simulink model "untitled"  (R2025a)
settings: Solver=VariableStepAuto  StartTime=0.0  StopTime=10.0  RelTol=1e-3
libraries: slpidlib x1
settings Model: Creator=MTMTAD006  LastModifiedBy=MTMTAD006

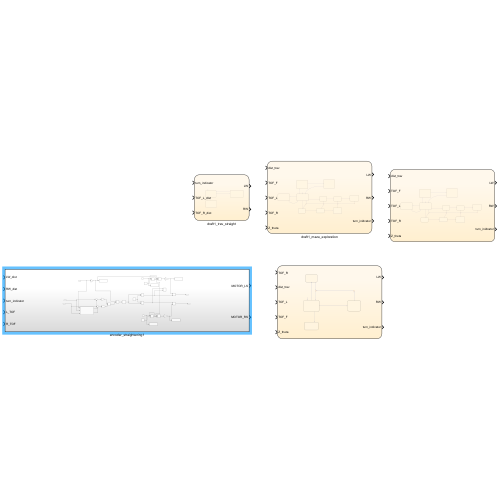
[thumbnail: Simulink's stored preview of the top-level diagram]
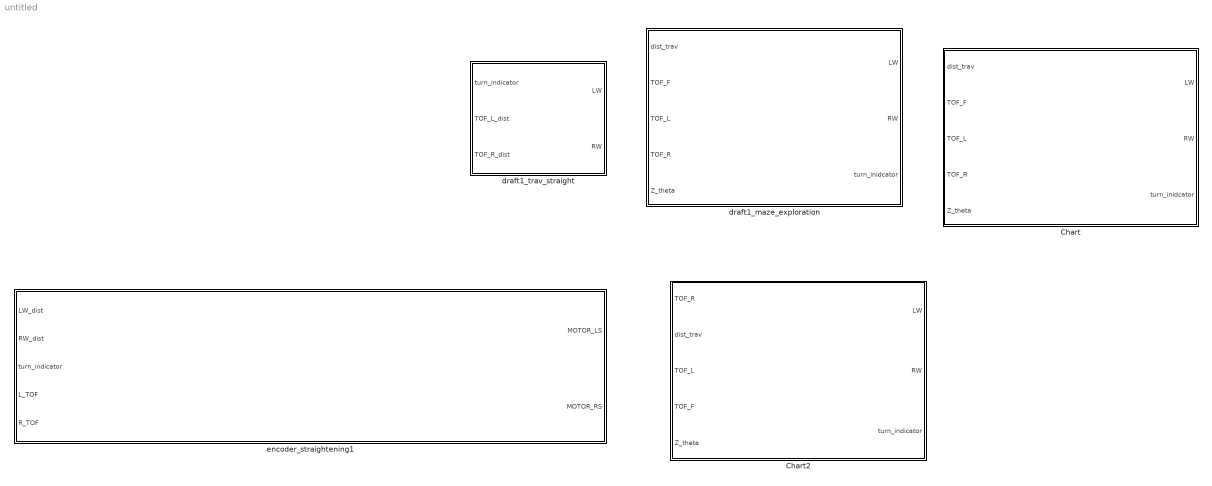
== system untitled ==
  Chart : Stateflow chart  TreatAsAtomicUnit=on
      settings: PortSchema="{\"entries\":[{\"content\":{\"sides\":[{\"content\":{\"connectorIds\":[\"In3\",\"In4\",\"In1\",\"In2\",\"In5\"]},\"type\":\"ConnectorPlacement.EquallySpacedRectSide\",\"uuid\":\"48a59af2-7c84-427a-8e2f-b10f2a044ed3\"},{\"content\":{\"connectorIds\":[\"Out1\",\"Out2\",\"Out3\"],\"side\":\"RIGHT\"},\"type\":\"ConnectorPlacement.EquallySpacedRectSide\",\"uuid\":\"ddb5ed95-9874-42e8-8fee-75458ccb7c53\"},{\"content\":{\"side\":\"TOP\"},\"type\":\"ConnectorPlacement.EquallySpacedRectSide\",\"uuid\":\"d57417fe-864c-49b1-b704-1964fc5ecc42\"}]},\"type\":\"ConnectorPlacement.EquallySpacedConnector\",\"uuid\":\"f24c4a6d-faf6-462a-ab68-e289d44b6927\"}],\"packageUris\":[\"http://schema.mathworks.com/mf0/Connector/R2020b\"],\"version\":\"1.0\"}"
  Chart2 : Stateflow chart  TreatAsAtomicUnit=on
      settings: PortSchema="{\"entries\":[{\"content\":{\"sides\":[{\"content\":{\"connectorIds\":[\"In2\",\"In3\",\"In1\",\"In4\",\"In5\"]},\"type\":\"ConnectorPlacement.EquallySpacedRectSide\",\"uuid\":\"48a59af2-7c84-427a-8e2f-b10f2a044ed3\"},{\"content\":{\"connectorIds\":[\"Out1\",\"Out2\",\"Out3\"],\"side\":\"RIGHT\"},\"type\":\"ConnectorPlacement.EquallySpacedRectSide\",\"uuid\":\"ddb5ed95-9874-42e8-8fee-75458ccb7c53\"},{\"content\":{\"side\":\"TOP\"},\"type\":\"ConnectorPlacement.EquallySpacedRectSide\",\"uuid\":\"d57417fe-864c-49b1-b704-1964fc5ecc42\"}]},\"type\":\"ConnectorPlacement.EquallySpacedConnector\",\"uuid\":\"f24c4a6d-faf6-462a-ab68-e289d44b6927\"}],\"packageUris\":[\"http://schema.mathworks.com/mf0/Connector/R2020b\"],\"version\":\"1.0\"}"
  draft1_maze_exploration : Stateflow chart  TreatAsAtomicUnit=on
      settings: PortSchema="{\"entries\":[{\"content\":{\"sides\":[{\"content\":{\"connectorIds\":[\"In3\",\"In4\",\"In1\",\"In2\",\"In5\"]},\"type\":\"ConnectorPlacement.EquallySpacedRectSide\",\"uuid\":\"48a59af2-7c84-427a-8e2f-b10f2a044ed3\"},{\"content\":{\"connectorIds\":[\"Out1\",\"Out2\",\"Out3\"],\"side\":\"RIGHT\"},\"type\":\"ConnectorPlacement.EquallySpacedRectSide\",\"uuid\":\"ddb5ed95-9874-42e8-8fee-75458ccb7c53\"},{\"content\":{\"side\":\"TOP\"},\"type\":\"ConnectorPlacement.EquallySpacedRectSide\",\"uuid\":\"d57417fe-864c-49b1-b704-1964fc5ecc42\"}]},\"type\":\"ConnectorPlacement.EquallySpacedConnector\",\"uuid\":\"f24c4a6d-faf6-462a-ab68-e289d44b6927\"}],\"packageUris\":[\"http://schema.mathworks.com/mf0/Connector/R2020b\"],\"version\":\"1.0\"}"
  draft1_trav_straight : Stateflow chart  TreatAsAtomicUnit=on
      settings: PortSchema="{\"entries\":[{\"content\":{\"sides\":[{\"content\":{\"connectorIds\":[\"In3\",\"In1\",\"In2\"]},\"type\":\"ConnectorPlacement.EquallySpacedRectSide\",\"uuid\":\"365a71ab-4b35-48e3-9778-a5038b9a912c\"},{\"content\":{\"connectorIds\":[\"Out1\",\"Out2\"],\"side\":\"RIGHT\"},\"type\":\"ConnectorPlacement.EquallySpacedRectSide\",\"uuid\":\"5548e51e-e574-4514-9ca7-4277d25c135b\"},{\"content\":{\"side\":\"TOP\"},\"type\":\"ConnectorPlacement.EquallySpacedRectSide\",\"uuid\":\"07b80b24-ee67-462d-94da-ddff32a3bc38\"}]},\"type\":\"ConnectorPlacement.EquallySpacedConnector\",\"uuid\":\"2b842345-bc9a-48c8-b3f2-d2787cfe54fa\"}],\"packageUris\":[\"http://schema.mathworks.com/mf0/Connector/R2020b\"],\"version\":\"1.0\"}"
  encoder_straightening1 : Subsystem

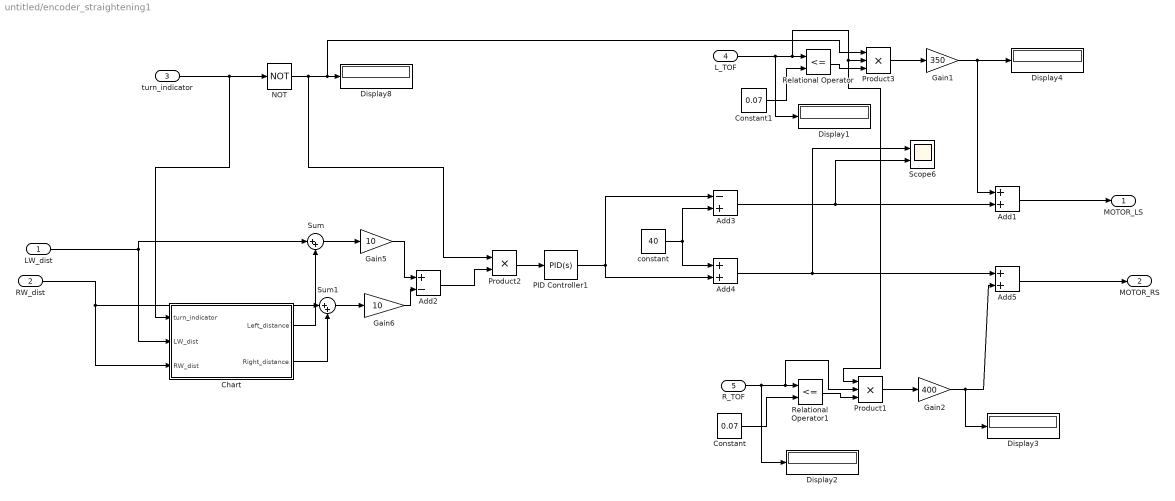
== system untitled/encoder_straightening1 ==
  LW_dist : Inport
  RW_dist : Inport  Port=2
  turn_indicator : Inport  Port=3
  L_TOF : Inport  Port=4
  R_TOF : Inport  Port=5
  Add1 : Sum
  Add2 : Sum  Inputs=+-
  Add3 : Sum  Inputs=-+
  Add4 : Sum
  Add5 : Sum
  Chart : Stateflow chart  TreatAsAtomicUnit=on
      settings: PortSchema="{\"entries\":[{\"content\":{\"sides\":[{\"content\":{\"connectorIds\":[\"In1\",\"In3\",\"In2\"]},\"type\":\"ConnectorPlacement.EquallySpacedRectSide\",\"uuid\":\"fc51768e-ed5b-46a0-b3fc-5b0af41a010d\"},{\"content\":{\"connectorIds\":[\"Out1\",\"Out2\"],\"side\":\"RIGHT\"},\"type\":\"ConnectorPlacement.EquallySpacedRectSide\",\"uuid\":\"30fd33ca-4b93-4317-9d26-1d1e6ba5d493\"},{\"content\":{\"side\":\"TOP\"},\"type\":\"ConnectorPlacement.EquallySpacedRectSide\",\"uuid\":\"029c60dd-f0f8-450d-b3c4-7fca568cb539\"}]},\"type\":\"ConnectorPlacement.EquallySpacedConnector\",\"uuid\":\"245ec1db-d65a-48a6-a1e3-28a0f03f23bc\"}],\"packageUris\":[\"http://schema.mathworks.com/mf0/Connector/R2020b\"],\"version\":\"1.0\"}"
  Constant : Constant  Value=0.07
  Constant1 : Constant  Value=0.07
  Display{1..4,8} (5 alike) : Display
  Gain1 : Gain  Gain=350
  Gain2 : Gain  Gain=400
  Gain5 : Gain  Gain=10
  Gain6 : Gain  Gain=10
  NOT : Logic  Operator=NOT  IconShape=distinctive  AllPortsSameDT=off  OutDataTypeStr=boolean
  PID Controller1 : slpidlib/PID Controller  Controller=PID  Form=Parallel  TimeDomain=Continuous-time  UseExternalTs=off  SampleTime=-1  IntegratorMethod=Forward Euler  FilterMethod=Forward Euler  ControllerParametersSource=internal  P=75  I=1  UseKiTs=off  D=0  UseExternalDerivativeSource=off  N=100  UseFilter=on  TunerSelectOption=Transfer Function Based (PID Tuner App)  InitialConditionSource=internal  InitialConditionForIntegrator=0  InitialConditionForFilter=0  DifferentiatorICPrevScaledInput=0  ExternalReset=none  TrackingMode=off  Kt=1  LimitOutput=off  SatLimitsSource=internal  UpperSaturationLimit=inf  LowerSaturationLimit=-inf  LinearizeAsGain=on  AntiWindupMode=none  Kb=1  LimitIntegrator=off  UpperIntegratorSaturationLimit=inf  LowerIntegratorSaturationLimit=-inf  POutMin=[]  POutMax=[]  IOutMin=[]  IOutMax=[]  DOutMin=[]  DOutMax=[]  NOutMin=[]  NOutMax=[]  SumOutMin=[]  SumOutMax=[]  SaturationOutMin=[]  SaturationOutMax=[]  PParamMin=[]  PParamMax=[]  IParamMin=[]  IParamMax=[]  DParamMin=[]  DParamMax=[]  NParamMin=[]  NParamMax=[]  KbParamMin=[]  KbParamMax=[]  KtParamMin=[]  KtParamMax=[]  KbOutMin=[]  KbOutMax=[]  KtOutMin=[]  KtOutMax=[]  IntegratorOutMin=[]  IntegratorOutMax=[]  FilterOutMin=[]  FilterOutMax=[]  SumI1OutMin=[]  SumI1OutMax=[]  SumI2OutMin=[]  SumI2OutMax=[]  SumI3OutMin=[]  SumI3OutMax=[]  SumI4OutMin=[]  SumI4OutMax=[]  SumDOutMin=[]  SumDOutMax=[]  DifferentiatorOutMin=[]  DifferentiatorOutMax=[]  FilterDiffOutCoefMin=[]  FilterDiffOutCoefMax=[]  ReciprocalOutMin=[]  ReciprocalOutMax=[]  SumDenOutMin=[]  SumDenOutMax=[]  SumNumOutMin=[]  SumNumOutMax=[]  DivideOutMin=[]  DivideOutMax=[]  UdiffTsProdOutMin=[]  UdiffTsProdOutMax=[]  NTsProdOutMin=[]  NTsProdOutMax=[]  UintegralTsProdOutMin=[]  UintegralTsProdOutMax=[]  UngainTsProdOutMin=[]  UngainTsProdOutMax=[]  ClampingZeroOutDataTypeStr=Inherit: Inherit via back propagation  ClampingZeroOutMin=[]  ClampingZeroOutMax=[]  FilterDenConstantOutDataTypeStr=Inherit: Inherit via back propagation  FilterDenConstantOutMin=[]  FilterDenConstantOutMax=[]  PCopyOutDataTypeStr=Inherit: Inherit via back propagation  PCopyOutMin=[]  PCopyOutMax=[]  NCopyOutDataTypeStr=Inherit: Inherit via back propagation  NCopyOutMin=[]  NCopyOutMax=[]  IntegratorContinuousStateAttributes=''  IntegratorStateMustResolveToSignalObject=off  IntegratorRTWStateStorageClass=Auto  FilterContinuousStateAttributes=''  FilterStateMustResolveToSignalObject=off  FilterRTWStateStorageClass=Auto  ParallelPVariant=InternalParameters  IdealPVariant=Disabled  IVariant=InternalParameters  DVariant=InternalParameters  IntegratorVariant=Continuous  SatVariant=Disabled  AWVariant=Passthrough  PCopyVariant=Disabled  TRVariant=Disabled  FdbkBlocksVariant=Forward  IdealPFdbkVariant=Disabled  SatFdbkVariant=Disabled  DerivativeFilterVariant=ContFilter  NVariant=InternalParameters  NCopyVariant=Disabled  FilterICVariant=InternalICsFilter  IntegratorICVariant=InternalICs  ExternalResetVariant=Disabled  TRSumVariant=Passthrough  SumFdbkVariant=Disabled  SumVariant=Sum_PID  TsampFilterVariant=InternalTs  TsampNgainVariant=Passthrough  TsampIntegralVariant=Disabled_SignalSpec  ExternalSaturationOutDataTypeStr=Inherit: Same as second input  DerivativeSourceVariant=ErrorSignal  PreIntVariant=InternalPreInt
  Product1 : Product  Inputs=3
  Product2 : Product
  Product3 : Product  Inputs=3
  Relational Operator : RelationalOperator  Operator=<=  OutDataTypeStr=boolean  RndMeth=Simplest  InputSameDT=off
  Relational Operator1 : RelationalOperator  Operator=<=  OutDataTypeStr=boolean  RndMeth=Simplest  InputSameDT=off
  Scope6 : Scope  NumInputPorts=2
      settings: ActiveDisplayYMinimum=-0.00015132169145948109  ActiveDisplayYMaximum=8.2179160600609662E-5  DataLoggingVariableName=ScopeData24
  Sum : Sum  Inputs=|++
  Sum1 : Sum  Inputs=|++
  constant : Constant  Value=40
  MOTOR_LS : Outport
  MOTOR_RS : Outport  Port=2
  wires:
  Gain1/1 -> Display4/1, Add1/1
  Gain2/1 -> Add5/2, Display3/1
  Add5/1 -> MOTOR_RS/1
  Product1/1 -> Gain2/1
  Add1/1 -> MOTOR_LS/1
  Product3/1 -> Gain1/1
  Constant1/1 -> Relational Operator/2
  Relational Operator/1 -> Product3/3
  Relational Operator1/1 -> Product1/3
  Constant/1 -> Relational Operator1/2
  R_TOF/1 -> Relational Operator1/1, Product1/2, Display2/1
  L_TOF/1 -> Relational Operator/1, Product3/2, Product1/1, Display1/1
  Chart/2(Right_distance) -> Sum1/2
  Sum1/1 -> Gain6/1
  Chart/1(Left_distance) -> Sum/2
  Sum/1 -> Gain5/1
  NOT/1 -> Display8/1, Product3/1, Product2/1
  RW_dist/1 -> Chart/2(RW_dist), Sum1/1
  LW_dist/1 -> Sum/1, Chart/3(LW_dist)
  turn_indicator/1 -> NOT/1, Chart/1(turn_indicator)
  Gain6/1 -> Add2/2
  PID Controller1/1 -> Add4/2, Add3/1
  Add2/1 -> Product2/2
  constant/1 -> Add4/1, Add3/2
  Product2/1 -> PID Controller1/1
  Add3/1 -> Add1/2, Scope6/2
  Gain5/1 -> Add2/1
  Add4/1 -> Scope6/1, Add5/1

== stateflow chart untitled/Chart ==
  settings: updateMethod=CONTINUOUS
  state Empty_rot_init
    entry:
    LW =0;
    RW = 0;
    theta = Z_theta;
    during:
    LW = 1;
    RW = -1;
  state Full_rot_init
    entry:
    LW =0.5;
    RW = 0.5;
    start_dist = dist_trav
  state INIT1
    entry:
    LW = 0.5;
    RW = 0.5;
    turn_inidcator = 0;
    start_dist = dist_trav;
  state INIT
    entry:
    LW = 1;
    RW = 1;
    turn_inidcator = 0;
  state Rotate
    entry:
    LW = 0;
    RW = 0;
    theta = Z_theta;
    during:
    RW = 1;
    LW = -1;
  state trn_left_init
    entry:
    start_dist = dist_trav;
    LW = 0;
    RW = 0;
  state Postion_robot
    entry:
    end_dist = start_dist + 0.13;
    LW = 0.5;
    RW =0.5;
  note: accutnign for false signale
  state Rotate1
    entry:
    LW = 0;
    RW = 0;
    theta = Z_theta;
    during:
    RW = -1;
    LW = 1;
  state trn_right_init1
    entry:
    start_dist = dist_trav;
    LW = 0;
    RW = 0;
  state Postion_robot1
    entry:
    end_dist = start_dist + 0.13;
    LW = 0.5;
    RW =0.5;
  Full_rot_init -> Empty_rot_init : [dist_trav >= 0.1]
  Empty_rot_init -> INIT : [Z_theta <= theta - pi]
  INIT -> Full_rot_init [order 4] : [TOF_R == 1 && TOF_L == 1 ]
  (default) -> INIT
  INIT -> INIT1 [order 1] : [TOF_F == 0]
  trn_left_init -> Postion_robot [order 2] : after(2,sec) [TOF_L == 0]
  Postion_robot -> Rotate [order 2] : [dist_trav >= end_dist]
  INIT -> trn_left_init [order 2] : [TOF_L == 0]
  INIT1 -> INIT : [TOF_F ==1 && TOF_L == 0 || TOF_R ==0]
  INIT -> trn_right_init1 [order 3] : [TOF_R == 0 ]
  (junction 20) -> INIT
  trn_left_init -> (junction 21) [order 1] : [TOF_L ==1 ]
  Postion_robot -> (junction 53) [order 1] : [TOF_L == 1]
  Rotate -> (junction 58) : [Z_theta >= pi/2 + theta ]
  (junction 58) -> (junction 53)
  (junction 53) -> (junction 21)
  (junction 21) -> (junction 20)
  trn_right_init1 -> (junction 20) [order 1] : [TOF_R == 1]
  Rotate1 -> (junction 53) : [Z_theta <= theta - pi/2]
  Postion_robot1 -> (junction 21) [order 1] : [TOF_R ==1 ]
  trn_right_init1 -> Postion_robot1 [order 2] : [TOF_R == 0]
  Postion_robot1 -> Rotate1 [order 2] : [dist_trav >= end_dist]
  data: TOF_L input; TOF_R input; LW output; RW output; dist_trav input; start_dist local; TOF_F input; end_dist local; Z_theta input; turn_inidcator output; theta local

== stateflow chart untitled/draft1_trav_straight ==
  state Turning_Right
    during:
    RW = 0.9;
    LW = 1;
  state Deafult
    entry:
    LW = 1;
    RW =1;
  state Turning_Left
    during:
    LW = 0.9;
    RW = 1;
  (default) -> Deafult
  Turning_Right -> Deafult : [TOF_R_dist == TOF_L_dist]
  Deafult -> Turning_Right [order 1] : [TOF_R_dist > TOF_L_dist && turn_indicator == 0]
  Turning_Left -> Deafult : [TOF_L_dist == TOF_R_dist]
  Deafult -> Turning_Left [order 2] : [TOF_L_dist > TOF_R_dist && turn_indicator == 0]
  data: TOF_L_dist input; TOF_R_dist input; LW output; RW output; turn_indicator input

== stateflow chart untitled/Chart2 ==
  settings: updateMethod=CONTINUOUS
  state Go_straight
    during:
    LW = 1;
    RW = 1;
  state Start
    entry:
    turn_indicator = 0;
  state Full_rotation
    entry:
    theta = Z_theta;
    turn_indicator = 1;
    during:
    LW = 1;
    RW =-1
  state Turn_right
    entry:
    theta = Z_theta
  Start -> Go_straight [order 2] : [TOF_L == 1 || TOF_R == 1 && TOF_F ==0]
  Go_straight -> (junction 107) : [TOF_F ==1 ]{LW =0; RW =0}
  (junction 103) -> (junction 107)
  (junction 107) -> Start
  Full_rotation -> (junction 103) : [Z_theta <= theta - pi && F == 0 ]
  (default) -> Start
  Start -> Full_rotation [order 1] : [TOF_L == 1 && TOF_R == 1 && TOF_F ==1]{LW =0; RW = 0 }
  Start -> Turn_right [order 3] : [TOF_R ==0]{LW = 0; RW =0}
  data: TOF_L input; TOF_R input; LW output; RW output; dist_trav input; start_dist local; TOF_F input; end_dist local; Z_theta input; turn_indicator output; theta local

== stateflow chart untitled/draft1_maze_exploration ==
  settings: updateMethod=CONTINUOUS
  state Empty_rot_init
    entry:
    LW =0;
    RW = 0;
    theta = Z_theta;
    during:
    LW = 1;
    RW = -1;
  state Full_rot_init
    entry:
    LW =0.5;
    RW = 0.5;
    start_dist = dist_trav
  state INIT1
    entry:
    LW = 0.5;
    RW = 0.5;
    turn_inidcator = 0;
    start_dist = dist_trav;
  state INIT
    entry:
    LW = 1;
    RW = 1;
    turn_inidcator = 0;
  state Rotate
    entry:
    RW =0;
    LW =0;
    theta = Z_theta;
    during:
    RW = 1;
    LW = -1;
  state trn_left_init
    entry:
    start_dist = dist_trav;
    LW = 0;
    RW = 0;
  state Postion_robot
    entry:
    end_dist = start_dist + 0.11;
    LW = 0.5;
    RW =0.5;
  note: accutnign for false signale
  state Rotate1
    entry:
    theta = Z_theta;
    during:
    RW = -1;
    LW = 1;
  state trn_right_init1
    entry:
    start_dist = dist_trav;
    LW = 0;
    RW = 0;
  state Postion_robot1
    entry:
    end_dist = start_dist + 0.11;
    LW = 0.5;
    RW =0.5;
  Full_rot_init -> Empty_rot_init : [dist_trav >= 0.1]
  Empty_rot_init -> INIT : [Z_theta <= theta - pi]
  INIT -> Full_rot_init [order 4] : [TOF_R == 1 && TOF_L == 1 ]
  (default) -> INIT
  INIT -> INIT1 [order 1] : [TOF_F == 0]
  trn_left_init -> Postion_robot [order 2] : after(2,sec) [TOF_L == 0]
  Postion_robot -> Rotate [order 2] : [dist_trav >= end_dist]
  INIT -> trn_left_init [order 2] : [TOF_L == 0]
  INIT1 -> INIT : [TOF_F ==1 && TOF_L == 0 || TOF_R ==0]
  INIT -> trn_right_init1 [order 3] : [TOF_R == 0 ]
  (junction 20) -> INIT
  trn_left_init -> (junction 21) [order 1] : [TOF_L ==1 ]
  Postion_robot -> (junction 53) [order 1] : [TOF_L == 1]
  Rotate -> (junction 58) : [Z_theta >= pi/2 + theta ]
  (junction 58) -> (junction 53)
  (junction 53) -> (junction 21)
  (junction 21) -> (junction 20)
  trn_right_init1 -> (junction 20) [order 1] : [TOF_R == 1]
  Rotate1 -> (junction 53) : [Z_theta <= theta - pi/2]
  Postion_robot1 -> (junction 21) [order 1] : [TOF_R ==1 ]
  trn_right_init1 -> Postion_robot1 [order 2] : [TOF_R == 0]
  Postion_robot1 -> Rotate1 [order 2] : [dist_trav >= end_dist]
  data: TOF_L input; TOF_R input; LW output; RW output; dist_trav input; start_dist local; TOF_F input; end_dist local; Z_theta input; turn_inidcator output; theta local

== stateflow chart untitled/encoder_straightening1/Chart ==
  state after_turn
    entry:
    during:
    if (LW_dist > RW_dist)
    Right_distance = difference;
    elseif (RW_dist > LW_dist)
    Left_distance =  difference;
    end
  state distance_corrcetion
    exit:
    difference = RW_dist - LW_dist;
    difference = abs(difference)
  (default) -> distance_corrcetion
  after_turn -> distance_corrcetion : [turn_indicator == 1]
  distance_corrcetion -> after_turn : [turn_indicator == 0]
  data: turn_indicator input; RW_dist input; Left_distance output; LW_dist input; Right_distance output; difference local
